simulink model "ES_video_newton_DSAS"  (R2020a)
settings: Solver=ode2  StartTime=0.0  StopTime=100  FixedStep=1/120  RelTol=1e-3
model workspace (MAT data in the model file):
  camera_rate = Simulink.Parameter
  camera_rate.Value = Simulink.data.Expression
  camera_rate.Value.ExpressionString = "qc_get_step_size * ceil(1/120 / qc_get_step_size)"
  camera_rate.DataType = 'auto'
  camera_rate.Dimensions = -1
  depth_rate = Simulink.Parameter
  depth_rate.Value = Simulink.data.Expression
  depth_rate.Value.ExpressionString = "qc_get_step_size * ceil(1/100 / qc_get_step_size)"
  depth_rate.DataType = 'auto'
  depth_rate.Dimensions = -1
values from neighbouring files (symbols this model uses):
  a_min = 0.01*[2;3;2;3;5;2]    [Parameters.m]
  amp = 0.5*[2;3;4;3;5;2]    [Parameters.m]
  d = 10*ones(6,1)    [Parameters.m]
  freq = 0.8*[0.0011;0.0054;0.0023;0.0037;0.0082;0.0041]*100    [Parameters.m]
  gain = (5*[30;20;21;10;15;20])    [Parameters.m]
  gain_amp = 0.001*[1;1;1;1;1;1]    [Parameters.m]
  IC = 1/2*diag([1 1 1 1 1 1])    [Parameters.m]
  r = 0.5    [Parameters.m]
  w_r = w * delta * 1    (= 0.01)    [Parameters.m]
undefined symbols (not defined in the file or in its folder): gcbh, JPEG, qc_get_step_size, video_display_show
libraries: quarc_library x13, simulink x3, powerlib_meascontrol x2, dspstat3 x1, visionsources x1
settings Model: PacingRate=8  ExtModeTrigDuration=10000  Creator=User  LastModifiedBy=user
settings SolverCC: PositivePriorityOrder=on
settings DataIOCC: ReturnWorkspaceOutputs=off
settings DebuggingCC: ParameterPrecisionLossMsg=none  ArithmeticOperatorsInVariantConditions=warning
settings HardwareCC: ProdBitPerLong=64  ProdLargestAtomicInteger=LongLong  ProdLargestAtomicFloat=Double  ProdLongLongMode=on  ProdHWDeviceType=ARM Compatible->ARM 64-bit (LP64)
settings SFSimCC: SimUseLocalCustomCode=off  CustomCodeUndefinedFunction=UseInterfaceOnly
settings RTWCC: Description=QUARC Linux Nvidia Target (QCar) Using Toolchain  SystemTargetFile=quarc_linux_nvidia.tlc  TemplateMakefile=quarc_default_tmf  RTWUseLocalCustomCode=off  Toolchain=QUARC linux_nvidia | gmake (64-bit Windows)  BuildConfiguration=Faster Runs
settings STFCustomTargetCC: TargetLangStandard=C99 (ISO)  ConcurrentExecutionCompliant=on  GRTInterface=on  UseToolchainInfoCompliant=on  SystemTargetFile=quarc_linux_nvidia.tlc
settings GRTTargetCC: ParMdlRefBuildCompliant=off  CompOptLevelCompliant=off  CombineOutputUpdateFcns=off  MatFileLogging=off  CPPClassGenCompliant=off  GRTInterface=on  ExtMode=on  ExtModeMexFile=quarc_comm  ExtModeMexArgs='-w -d /tmp -uri %u', 'tcpip://192.168.2.11:17001'

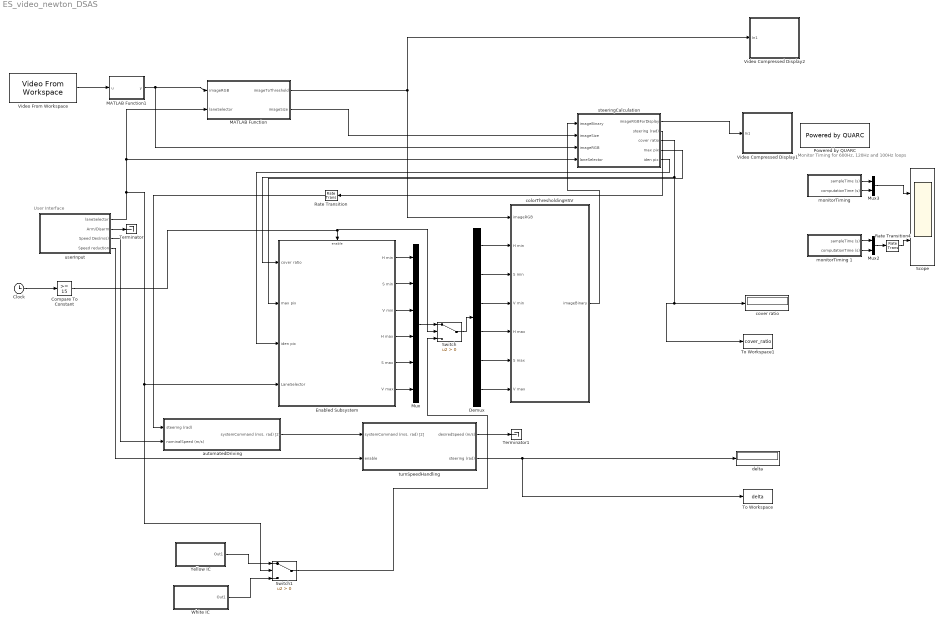
== system ES_video_newton_DSAS ==
  note: User Interface
  note: Monitor Timing for 600Hz, 120Hz and 100Hz loops
  Clock : Clock
  Compare To Constant : simulink/Logic and Bit Operations/Compare To Constant  relop=>=  const=15  OutDataTypeStr=boolean
  Demux : Demux  Outputs=6
  Enabled Subsystem : Subsystem  TreatAsAtomicUnit=on
  MATLAB Function : MATLAB Function  TreatAsAtomicUnit=on
  MATLAB Function1 : MATLAB Function  TreatAsAtomicUnit=on
  Mux : Mux  Inputs=6
  Mux2 : Mux  Inputs=2
  Mux3 : Mux  Inputs=2
  Powered by QUARC : quarc_library/Logos/Powered by QUARC
  Rate Transition : RateTransition
  Rate Transition4 : RateTransition
  Scope : Scope  NumInputPorts=2
  Switch : Switch  Criteria=u2 > Threshold
  Switch1 : Switch  Criteria=u2 > Threshold
  Terminator : Terminator
  Terminator1 : Terminator
  To Workspace : ToWorkspace  VariableName=delta  SaveFormat=Structure With Time  SampleTime=-1
  To Workspace1 : ToWorkspace  VariableName=cover_ratio  SaveFormat=Structure With Time  SampleTime=-1
      settings: Save2DSignal=2-D array (concatenate along first dimension)
  Video Compressed Display1 : Subsystem  LoadFcn=set_param(gcbh, 'UserData', gcb);  StartFcn=video_display_show([gcb, '/Video Display'], 'add', gcb);  mask(Video Compressed Display){algorithm=JPEG, quality=50, sample_time=-1, use_hardware=on}
      mask prompts: algorithm "Compression algorithm:"; quality "Compression quality (0-100):"; sample_time "Sample time (seconds):"; use_hardware "Use hardware acceleration for video display"
      mask help: Displays a video stream on the host, using compression to minimize bandwidth.
      mask init:
      | qc_set_display('Video\nCompressed\nDisplay');
      settings: UndoDeleteFcn=set_param(gcbh, 'UserData', gcb);  OpenFcn=video_display_show([gcb, '/Video Display'], 'show', gcb);  PreDeleteFcn=video_display_show([gcb, '/Video Display'], 'delete');
      settings: CopyFcn=|
      | set_param(gcbh, 'UserData', gcb);
      | set_param(gcbh, 'LinkStatus', 'none');
      settings: NameChangeFcn=|
      | video_display_show([get_param(gcbh, 'UserData'), '/Video Display'], 'rename', [gcb, '/Video Display']);
      | video_display_show([gcb, '/Video Display'], 'add', gcb);
      | set_param(gcbh, 'UserData', gcb);
      mask Help: web(qc_get_block_help_path(gcb));
      mask TypeOptions algorithm: Image Compress/algorithm
      mask TypeOptions quality: Image Compress/quality
      mask TypeOptions sample_time: Video Display/sample_time
      mask TypeOptions use_hardware: Video Display/use_hardware
      mask Display:
      | patch([0.98591 0.98591 0.62618 0.59072 0.56147   0.536   0.536  0.5441 0.56912 0.59207 0.60881 0.62276 0.63527 0.64364  0.6485  0.6485 0.64706 0.64499 0.63662 0.62411 0.61232 0.59837 0.58307 0.56147   0.536   0.536  0.5441  0.5747 0.60953 0.63662 0.67001  0.7034 0.72851 0.75425 0.77927 0.80294 0.82454 0.84119 0.85865 0.87395 0.88574 0.89339  0.8969 0.89969 0.89969 0.89267  0.8816 0.87044 0.85649  0.8384 0.81824 0.80294 0.78764 0.77513 0.76676 0.75776 0.76397 0.77513 0.79178 0.80987 0.82796 0.84326 0.86207 0.98528],[0.18689 0.05522 0.05522 0.05171 0.05171    0.05 0.18338 0.18338 0.19148 0.20435 0.22298 0.24863 0.28589 0.33125 0.38138 0.55139 0.59801 0.63761 0.68189 0.72149 0.74939 0.76694 0.77855 0.79367 0.79952 0.92768 0.92768 0.92768 0.92417 0.92066 0.91364  0.9032 0.89384 0.88106 0.86594 0.85073 0.82634 0.80537 0.77855 0.74363 0.70403 0.65858 0.61079 0.59099 0.41513 0.37202 0.31847 0.29048 0.25556 0.23342  0.2102 0.19382 0.18221 0.17285 0.16943 0.16124  0.1589 0.16241 0.16709 0.17168  0.1787 0.18221 0.18689 0.18689],[0.9,0.90,0.91])
      | patch([0.536 0.52601 0.46823 0.44528 0.41603 0.39101 0.35555 0.33116 0.31451 0.29291  0.2804 0.26717 0.25322 0.23999 0.22406 0.20732 0.19337 0.17528 0.15935 0.14396 0.13217 0.11759 0.10922 0.10085 0.09671 0.09392 0.09041 0.08906 0.08906 0.09464  0.0995 0.10778 0.11894 0.13145 0.14675 0.16349 0.17672 0.19409 0.20732 0.22406 0.23999 0.26159 0.27833 0.29849 0.31793 0.33602 0.35411 0.37085 0.39245 0.41603   0.536   0.536 0.53159 0.46409   0.446 0.42026 0.39587 0.37571 0.36113 0.34925 0.34088 0.33809 0.33809 0.34088 0.34583 0.35627 0.36392 0.38129 0.39587 0.41117 0.42719 0.44672  0.4676 0.48353 0.48353 0.52394   0.536],[0.05 0.04829 0.04712 0.04712 0.04829 0.05063 0.05405 0.05873 0.06107 0.06692 0.07043 0.07619 0.08087 0.08672 0.09482 0.10652 0.11696 0.13325  0.1508 0.17168 0.19499 0.22415 0.25439 0.28472 0.31379 0.35456 0.38489 0.41513 0.58055 0.63878 0.68774 0.72149 0.75641 0.78089 0.80537 0.82859 0.84029 0.85658 0.86594 0.87404  0.8834 0.89267 0.90086 0.90788 0.91247 0.91832 0.92066   0.923 0.92651 0.92768 0.92768 0.79952 0.79952 0.79952 0.79718 0.78899 0.77153 0.75056 0.72149 0.68072 0.62249  0.5549 0.41396 0.37085 0.33242 0.28121 0.25205 0.22181 0.20552 0.19499 0.18572 0.18221 0.17753 0.17636 0.17753  0.1787  0.1787],[0.9,0.90,0.91])
      | disp('Video\nCompressed\nDisplay');
  Video Compressed Display2 : Subsystem  LoadFcn=set_param(gcbh, 'UserData', gcb);  StartFcn=video_display_show([gcb, '/Video Display'], 'add', gcb);  mask(Video Compressed Display){algorithm=JPEG, quality=50, sample_time=-1, use_hardware=on}
      mask prompts: algorithm "Compression algorithm:"; quality "Compression quality (0-100):"; sample_time "Sample time (seconds):"; use_hardware "Use hardware acceleration for video display"
      mask help: Displays a video stream on the host, using compression to minimize bandwidth.
      mask init:
      | qc_set_display('Video\nCompressed\nDisplay');
      settings: UndoDeleteFcn=set_param(gcbh, 'UserData', gcb);  OpenFcn=video_display_show([gcb, '/Video Display'], 'show', gcb);  PreDeleteFcn=video_display_show([gcb, '/Video Display'], 'delete');
      settings: CopyFcn=|
      | set_param(gcbh, 'UserData', gcb);
      | set_param(gcbh, 'LinkStatus', 'none');
      settings: NameChangeFcn=|
      | video_display_show([get_param(gcbh, 'UserData'), '/Video Display'], 'rename', [gcb, '/Video Display']);
      | video_display_show([gcb, '/Video Display'], 'add', gcb);
      | set_param(gcbh, 'UserData', gcb);
      mask Help: web(qc_get_block_help_path(gcb));
      mask TypeOptions algorithm: Image Compress/algorithm
      mask TypeOptions quality: Image Compress/quality
      mask TypeOptions sample_time: Video Display/sample_time
      mask TypeOptions use_hardware: Video Display/use_hardware
      mask Display:
      | patch([0.98591 0.98591 0.62618 0.59072 0.56147   0.536   0.536  0.5441 0.56912 0.59207 0.60881 0.62276 0.63527 0.64364  0.6485  0.6485 0.64706 0.64499 0.63662 0.62411 0.61232 0.59837 0.58307 0.56147   0.536   0.536  0.5441  0.5747 0.60953 0.63662 0.67001  0.7034 0.72851 0.75425 0.77927 0.80294 0.82454 0.84119 0.85865 0.87395 0.88574 0.89339  0.8969 0.89969 0.89969 0.89267  0.8816 0.87044 0.85649  0.8384 0.81824 0.80294 0.78764 0.77513 0.76676 0.75776 0.76397 0.77513 0.79178 0.80987 0.82796 0.84326 0.86207 0.98528],[0.18689 0.05522 0.05522 0.05171 0.05171    0.05 0.18338 0.18338 0.19148 0.20435 0.22298 0.24863 0.28589 0.33125 0.38138 0.55139 0.59801 0.63761 0.68189 0.72149 0.74939 0.76694 0.77855 0.79367 0.79952 0.92768 0.92768 0.92768 0.92417 0.92066 0.91364  0.9032 0.89384 0.88106 0.86594 0.85073 0.82634 0.80537 0.77855 0.74363 0.70403 0.65858 0.61079 0.59099 0.41513 0.37202 0.31847 0.29048 0.25556 0.23342  0.2102 0.19382 0.18221 0.17285 0.16943 0.16124  0.1589 0.16241 0.16709 0.17168  0.1787 0.18221 0.18689 0.18689],[0.9,0.90,0.91])
      | patch([0.536 0.52601 0.46823 0.44528 0.41603 0.39101 0.35555 0.33116 0.31451 0.29291  0.2804 0.26717 0.25322 0.23999 0.22406 0.20732 0.19337 0.17528 0.15935 0.14396 0.13217 0.11759 0.10922 0.10085 0.09671 0.09392 0.09041 0.08906 0.08906 0.09464  0.0995 0.10778 0.11894 0.13145 0.14675 0.16349 0.17672 0.19409 0.20732 0.22406 0.23999 0.26159 0.27833 0.29849 0.31793 0.33602 0.35411 0.37085 0.39245 0.41603   0.536   0.536 0.53159 0.46409   0.446 0.42026 0.39587 0.37571 0.36113 0.34925 0.34088 0.33809 0.33809 0.34088 0.34583 0.35627 0.36392 0.38129 0.39587 0.41117 0.42719 0.44672  0.4676 0.48353 0.48353 0.52394   0.536],[0.05 0.04829 0.04712 0.04712 0.04829 0.05063 0.05405 0.05873 0.06107 0.06692 0.07043 0.07619 0.08087 0.08672 0.09482 0.10652 0.11696 0.13325  0.1508 0.17168 0.19499 0.22415 0.25439 0.28472 0.31379 0.35456 0.38489 0.41513 0.58055 0.63878 0.68774 0.72149 0.75641 0.78089 0.80537 0.82859 0.84029 0.85658 0.86594 0.87404  0.8834 0.89267 0.90086 0.90788 0.91247 0.91832 0.92066   0.923 0.92651 0.92768 0.92768 0.79952 0.79952 0.79952 0.79718 0.78899 0.77153 0.75056 0.72149 0.68072 0.62249  0.5549 0.41396 0.37085 0.33242 0.28121 0.25205 0.22181 0.20552 0.19499 0.18572 0.18221 0.17753 0.17636 0.17753  0.1787  0.1787],[0.9,0.90,0.91])
      | disp('Video\nCompressed\nDisplay');
  Video From Workspace : visionsources/Video From Workspace  signal=led  Ts=1/12  finalout=Obsolete  finaloutActive=Setting to zero  imagePorts=One multidimensional signal  OutPortLabels=R|G|B
      settings: SourceProductBaseCode=VP
  White IC : Subsystem
  Yellow IC : Subsystem
  automatedDriving : Subsystem
  colorThresholdingHSV : Subsystem
  cover ratio : Display
  "delta " : Display
  "monitorTiming " : Subsystem
  monitorTiming 1 : Subsystem
  steeringCalculation : Subsystem
  turnSpeedHandling : Subsystem
  userInput : Subsystem
  wires:
  userInput/4(Speed reduction) -> turnSpeedHandling/2(enable)
  automatedDriving/1("systemCommand (m/s, rad) [2]") -> turnSpeedHandling/1("systemCommand (m/s, rad) [2]")
  Rate Transition/1 -> automatedDriving/1(steering (rad))
  monitorTiming 1/2(computationTime (s)) -> Mux2/2
  monitorTiming 1/1(sampleTime (s)) -> Mux2/1
  "monitorTiming "/2(computationTime (s)) -> Mux3/2
  "monitorTiming "/1(sampleTime (s)) -> Mux3/1
  Mux2/1 -> Rate Transition4/1
  Mux3/1 -> Scope/1
  Rate Transition4/1 -> Scope/2
  colorThresholdingHSV/1(imageBinary) -> steeringCalculation/1(imageBinary)
  steeringCalculation/1(imageRGBForDisplay) -> Video Compressed Display1/1(In1)
  MATLAB Function/1(imageToThreshold) -> Video Compressed Display2/1(In1), colorThresholdingHSV/1(imageRGB)
  MATLAB Function/2(imageSize) -> steeringCalculation/2(imageSize)
  userInput/3(Speed Des(m/s)) -> automatedDriving/2(nominalSpeed (m/s))
  steeringCalculation/2(steering (rad)) -> Rate Transition/1
  Video From Workspace/1 -> MATLAB Function1/1(u)
  userInput/2(Arm/Disarm) -> Terminator/1
  MATLAB Function1/1(y) -> steeringCalculation/3(imageRGB), MATLAB Function/1(imageRGB)
  turnSpeedHandling/2(steering (rad)) -> To Workspace/1, "delta "/1
  steeringCalculation/3("cover ratio ") -> Enabled Subsystem/1(cover ratio), To Workspace1/1, cover ratio/1
  turnSpeedHandling/1(desiredSpeed (m/s)) -> Terminator1/1
  Clock/1 -> Compare To Constant/1
  Compare To Constant/1 -> Switch/2, Enabled Subsystem/Enable
  Enabled Subsystem/1(H min) -> Mux/1
  Enabled Subsystem/2(S min) -> Mux/2
  Enabled Subsystem/3(V min) -> Mux/3
  Enabled Subsystem/4(H max) -> Mux/4
  Enabled Subsystem/5(S max) -> Mux/5
  Enabled Subsystem/6(V max) -> Mux/6
  Mux/1 -> Switch/1
  Demux/6 -> colorThresholdingHSV/7(V max)
  Switch/1 -> Demux/1
  Demux/1 -> colorThresholdingHSV/2(H min)
  Demux/2 -> colorThresholdingHSV/3(S min)
  Demux/3 -> colorThresholdingHSV/4(V min)
  Demux/4 -> colorThresholdingHSV/5(H max)
  Demux/5 -> colorThresholdingHSV/6(S max)
  steeringCalculation/4(max pix) -> Enabled Subsystem/2(max pix)
  steeringCalculation/5(iden pix) -> Enabled Subsystem/3(iden pix)
  White IC/1(Out1) -> Switch1/3
  Yellow IC/1(Out1) -> Switch1/1
  Switch1/1 -> Switch/3
  userInput/1(laneSelector) -> Enabled Subsystem/4(LaneSelector), Switch1/2, MATLAB Function/2(laneSelector), steeringCalculation/4(laneSelector)

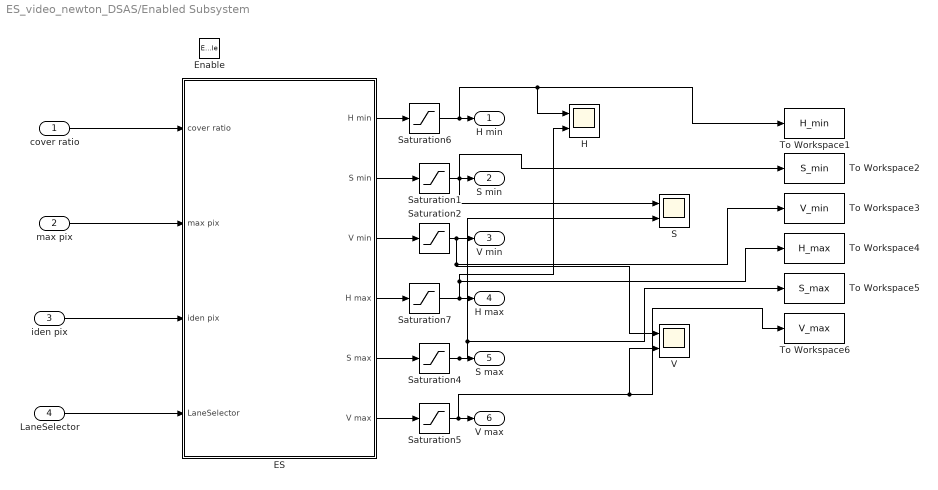
== system ES_video_newton_DSAS/Enabled Subsystem ==
  cover ratio : Inport
  max pix : Inport  Port=2
  iden pix : Inport  Port=3
  LaneSelector : Inport  Port=4
  Enable : EnablePort
  ES : Subsystem
  H : Scope  NumInputPorts=2
  S : Scope  NumInputPorts=2
  Saturation{1..2,4..7} (6 alike) : Saturate  UpperLimit=255  LowerLimit=0
  To Workspace1 : ToWorkspace  VariableName=H_min  SaveFormat=Timeseries  SampleTime=-1
      settings: Save2DSignal=2-D array (concatenate along first dimension)
  To Workspace2 : ToWorkspace  VariableName=S_min  SaveFormat=Timeseries  SampleTime=-1
      settings: Save2DSignal=2-D array (concatenate along first dimension)
  To Workspace3 : ToWorkspace  VariableName=V_min  SaveFormat=Timeseries  SampleTime=-1
      settings: Save2DSignal=2-D array (concatenate along first dimension)
  To Workspace4 : ToWorkspace  VariableName=H_max  SaveFormat=Timeseries  SampleTime=-1
      settings: Save2DSignal=2-D array (concatenate along first dimension)
  To Workspace5 : ToWorkspace  VariableName=S_max  SaveFormat=Timeseries  SampleTime=-1
      settings: Save2DSignal=2-D array (concatenate along first dimension)
  To Workspace6 : ToWorkspace  VariableName=V_max  SaveFormat=Timeseries  SampleTime=-1
      settings: Save2DSignal=2-D array (concatenate along first dimension)
  V : Scope  NumInputPorts=2
  H min : Outport  VectorParamsAs1DForOutWhenUnconnected=off
  S min : Outport  Port=2  VectorParamsAs1DForOutWhenUnconnected=off
  V min : Outport  Port=3  VectorParamsAs1DForOutWhenUnconnected=off
  H max : Outport  Port=4  VectorParamsAs1DForOutWhenUnconnected=off
  S max : Outport  Port=5  VectorParamsAs1DForOutWhenUnconnected=off
  V max : Outport  Port=6  VectorParamsAs1DForOutWhenUnconnected=off
  wires:
  cover ratio/1 -> ES/1("cover ratio ")
  ES/2(S min) -> Saturation1/1
  ES/3(V min) -> Saturation2/1
  ES/5(S max) -> Saturation4/1
  ES/6(V max) -> Saturation5/1
  max pix/1 -> ES/2("max pix ")
  iden pix/1 -> ES/3(iden pix)
  Saturation2/1 -> To Workspace3/1, V/1, V min/1
  Saturation5/1 -> To Workspace6/1, V/2, V max/1
  ES/4(H max) -> Saturation7/1
  Saturation1/1 -> To Workspace2/1, S min/1, S/1
  Saturation4/1 -> To Workspace5/1, S/2, S max/1
  ES/1(H min) -> Saturation6/1
  Saturation6/1 -> To Workspace1/1, H/1, H min/1
  Saturation7/1 -> To Workspace4/1, H/2, H max/1
  LaneSelector/1 -> ES/4(LaneSelector)

== system ES_video_newton_DSAS/Video Compressed Display1 ==
  In1 : Inport
  Channel : quarc_library/Signal Routing/Channel  channel=0  buffer_size=1
  Image Compress : quarc_library/Image Processing/Generic/Image Compress  algorithm=JPEG  source=Internal dialog parameter  quality=quality  output_dim=-1
  Video Display : quarc_library/Multimedia/Video Display  Tag=ES_video_newton_DSAS/Video Compressed Display1/Video Display  sample_time=sample_time  use_hardware=on
  wires:
  Channel/1 -> Video Display/1
  In1/1 -> Image Compress/1
  Image Compress/1 -> Channel/1

== system ES_video_newton_DSAS/Video Compressed Display2 ==
  In1 : Inport
  Channel : quarc_library/Signal Routing/Channel  channel=1  buffer_size=1
  Image Compress : quarc_library/Image Processing/Generic/Image Compress  algorithm=JPEG  source=Internal dialog parameter  quality=quality  output_dim=-1
  Video Display : quarc_library/Multimedia/Video Display  Tag=ES_video_newton_DSAS/Video Compressed Display2/Video Display  sample_time=sample_time  use_hardware=on
  wires:
  Image Compress/1 -> Channel/1
  In1/1 -> Image Compress/1
  Channel/1 -> Video Display/1

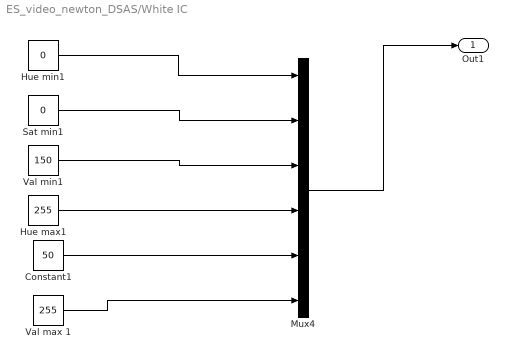
== system ES_video_newton_DSAS/White IC ==
  Constant1 : Constant  Value=50
  Hue max1 : Constant  Value=255
  Hue min1 : Constant  Value=0
  Mux4 : Mux  Inputs=6
  Sat min1 : Constant  Value=0
  Val max 1 : Constant  Value=255
  Val min1 : Constant  Value=150
  Out1 : Outport  VectorParamsAs1DForOutWhenUnconnected=off
  wires:
  Mux4/1 -> Out1/1
  Constant1/1 -> Mux4/5
  Sat min1/1 -> Mux4/2
  Hue min1/1 -> Mux4/1
  Val min1/1 -> Mux4/3
  Val max 1/1 -> Mux4/6
  Hue max1/1 -> Mux4/4

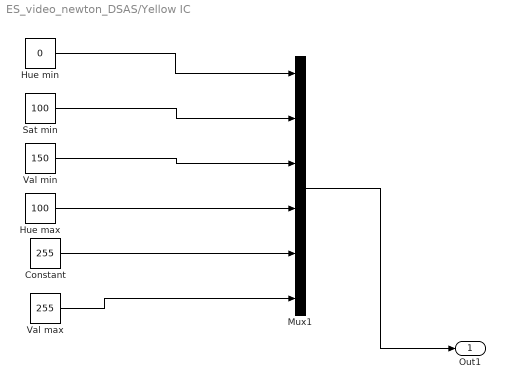
== system ES_video_newton_DSAS/Yellow IC ==
  Constant : Constant  Value=255
  Hue max : Constant  Value=100
  Hue min : Constant  Value=0
  Mux1 : Mux  Inputs=6
  Sat min : Constant  Value=100
  "Val max " : Constant  Value=255
  Val min : Constant  Value=150
  Out1 : Outport  VectorParamsAs1DForOutWhenUnconnected=off
  wires:
  Hue max/1 -> Mux1/4
  Val min/1 -> Mux1/3
  Hue min/1 -> Mux1/1
  "Val max "/1 -> Mux1/6
  Mux1/1 -> Out1/1
  Constant/1 -> Mux1/5
  Sat min/1 -> Mux1/2

== system ES_video_newton_DSAS/automatedDriving ==
  note: Automated-Driving Module:
      |
      | This subsystem provides a speed setpoint based on obstacles detected, while also transitioning rates. The speed setpoint is set to the nominal speed, and scales down linearly to zero depending on nominal tracking distance and stop distance.
      |
      | Inputs:
      | obstacleDistance (m) n/a : Distance to obstacle in meters
      | steering (rad) n/a : Steering output from image processing in radians
      | nominalSpeed (m/s) n/a : Desired speed setpoint
      |
      | Outputs:
      | systemCommand (m/s, rad) n/a : Commands representing speed setpoint and steering
      |
      | Usage:
      | 1. Set the Nominal Tracking distance. The speed setpoint will start decreasing if the obstacle distance is less than this threshold.
      | 2. Set the Stop Distance. The speed setpoint will scale down to 0 when the the obstacle distance reaches this threshold.
  steering (rad) : Inport
  nominalSpeed (m/s) : Inport  Port=2
  Mux1 : Mux  Inputs=2
  "systemCommand (m/s, rad) [2]" : Outport  VectorParamsAs1DForOutWhenUnconnected=off
  wires:
  nominalSpeed (m/s)/1 -> Mux1/1  "nominal speed (m/s)"
  steering (rad)/1 -> Mux1/2
  Mux1/1 -> "systemCommand (m/s, rad) [2]"/1

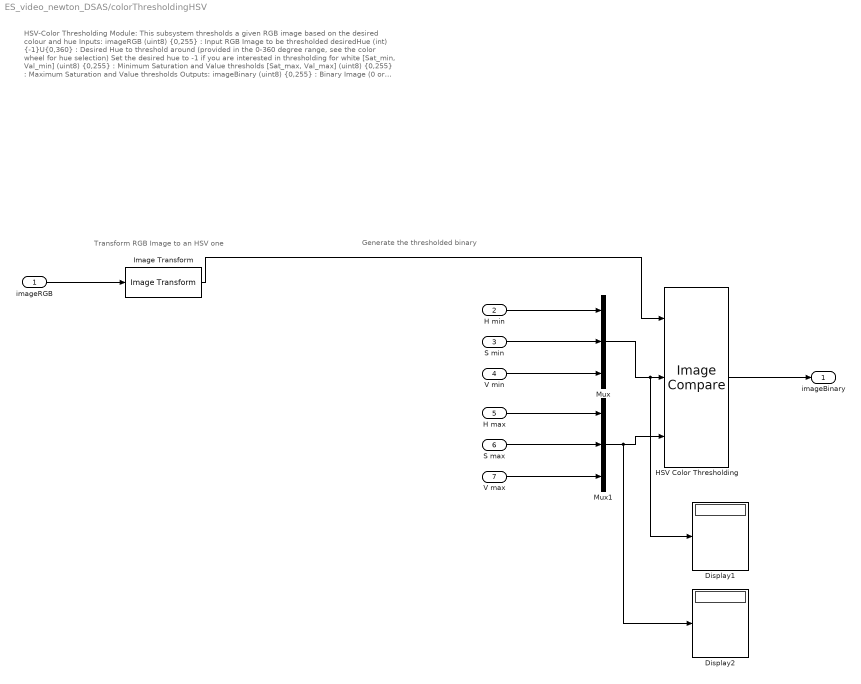
== system ES_video_newton_DSAS/colorThresholdingHSV ==
  note: HSV-Color Thresholding Module:
      |
      | This subsystem thresholds a given RGB image based on the desired colour and hue
      |
      | Inputs:
      | imageRGB (uint8) {0,255} : Input RGB Image to be thresholded
      | desiredHue (int) {-1}U{0,360} : Desired Hue to threshold around (provided in the 0-360 degree range, see the color wheel for hue selection)
      | Set the desired hue to -1 if you are interested in thresholding for white
      | [Sat_min, Val_min] (uint8) {0,255} : Minimum Saturation and Value thresholds
      | [Sat_max, Val_max] (uint8) {0,255} : Maximum Saturation and Value thresholds
      |
      | Outputs:
      | imageBinary (uint8) {0,255} : Binary Image (0 or 255 and no other value) representing the thresholding output
      |
      | Usage:
      | This module can be used when you are interested in thresholding for a certain hue regardless of the luminance. Compared to RGB thresholding which does not work well when the lighting conditions vary, HSV thresholding will correctly threshold for a hue (color) and allow you to specify a broad range of illuminance via the saturation and value thresholds. To broaden the range of hues accepted in the thresholding block, increase the Hue Threshold parameter.
  note: Transform RGB Image to an HSV one
  note: Generate the thresholded binary
  imageRGB : Inport
  H min : Inport  Port=2
  S min : Inport  Port=3
  V min : Inport  Port=4
  H max : Inport  Port=5
  S max : Inport  Port=6
  V max : Inport  Port=7
  Display1 : Display
  Display2 : Display
  HSV Color Thresholding : quarc_library/Image Processing/Generic/Image Compare  output_type=Combined (one HxW output)  source=External input ports  r_comparison=min <= pixel and pixel <= max with wrapping  r_minimum=30  r_maximum=70  g_comparison=min <= pixel and pixel <= max with wrapping  g_minimum=60  g_maximum=100  b_comparison=min <= pixel and pixel <= max with wrapping  b_minimum=40  b_maximum=80
      settings: SourceProductName=QUARC Targets
  Image Transform : quarc_library/Image Processing/Generic/Image Transform  algorithm=RGB to HSV  color_theme=KRYGCBMW  min_pixel=0  max_pixel=4000  focal_length=308  principal_point=[334 262]  radial_coeffs=[-0.3129 0.0907]  tangential_coeffs=[]  extrapolated_pixel=0  interpolation=nearest  row_coords=0  column_coords=0  output_height=480  output_width=640  angle=0  origin=[320 240]  output_origin=[320 240]
      settings: AttributesFormatString=(%<algorithm>)  SourceProductName=QUARC Targets
  Mux : Mux  Inputs=3
  Mux1 : Mux  Inputs=3
  imageBinary : Outport  VectorParamsAs1DForOutWhenUnconnected=off
  wires:
  Image Transform/1 -> HSV Color Thresholding/1
  imageRGB/1 -> Image Transform/1
  HSV Color Thresholding/1 -> imageBinary/1
  Mux/1 -> Display1/1, HSV Color Thresholding/2
  Mux1/1 -> Display2/1, HSV Color Thresholding/3
  S min/1 -> Mux/2
  H max/1 -> Mux1/1
  S max/1 -> Mux1/2
  V max/1 -> Mux1/3
  H min/1 -> Mux/1
  V min/1 -> Mux/3

== system ES_video_newton_DSAS/monitorTiming  ==
  note: moniorTiming Module:
      |
      | This subsystem outputs the sample time and computation time of the model.
      |
      | Outputs:
      | sampleTime (s) n/a : Sample time (unfiltered and filtered) in seconds.
      | computationTime (s) n/a : Computation time (unfiltered and filtered) in seconds.
      |
      | Usage:
      | Compare the Sample Time (s) output to a constant (qc_get_step_size) to monitor whether or not the desired sample time is being achieved. The Computation Time (s) values should be lower than the corresponding sample time value to ensure that the solver has enough time per time step.
  note: Timing Performance
  Computation Time : quarc_library/Sources/Time/Computation Time  sample_time=qc_get_step_size  use_model=on  use_cpu_time=off
  Constant : Constant  Value=qc_get_step_size  SampleTime=-1
  Mux : Mux  Inputs=2
  Sample Time : quarc_library/Sources/Time/Sample Time  Priority=-99  sample_time=qc_get_step_size
  sampleTime (s) : Outport  VectorParamsAs1DForOutWhenUnconnected=off
  computationTime (s) : Outport  Port=2  VectorParamsAs1DForOutWhenUnconnected=off
  wires:
  Computation Time/1 -> computationTime (s)/1
  Constant/1 -> Mux/2
  Sample Time/1 -> Mux/1
  Mux/1 -> sampleTime (s)/1

== system ES_video_newton_DSAS/monitorTiming 1 ==
  note: Timing Performance
  note: moniorTiming Module:
      |
      | This subsystem outputs the sample time and computation time of the model.
      |
      | Outputs:
      | sampleTime (s) n/a : Sample time (unfiltered and filtered) in seconds.
      | computationTime (s) n/a : Computation time (unfiltered and filtered) in seconds.
      |
      | Usage:
      | Compare the Sample Time (s) output to a constant (qc_get_step_size) to monitor whether or not the desired sample time is being achieved. The Computation Time (s) values should be lower than the corresponding sample time value to ensure that the solver has enough time per time step.
  Computation Time : quarc_library/Sources/Time/Computation Time  sample_time=camera_rate  use_model=on  use_cpu_time=off
  Constant : Constant  Value=camera_rate  SampleTime=camera_rate
  Mux : Mux  Inputs=2
  Sample Time : quarc_library/Sources/Time/Sample Time  Priority=-99  sample_time=camera_rate
  sampleTime (s) : Outport  VectorParamsAs1DForOutWhenUnconnected=off
  computationTime (s) : Outport  Port=2  VectorParamsAs1DForOutWhenUnconnected=off
  wires:
  Computation Time/1 -> computationTime (s)/1
  Mux/1 -> sampleTime (s)/1
  Sample Time/1 -> Mux/1
  Constant/1 -> Mux/2

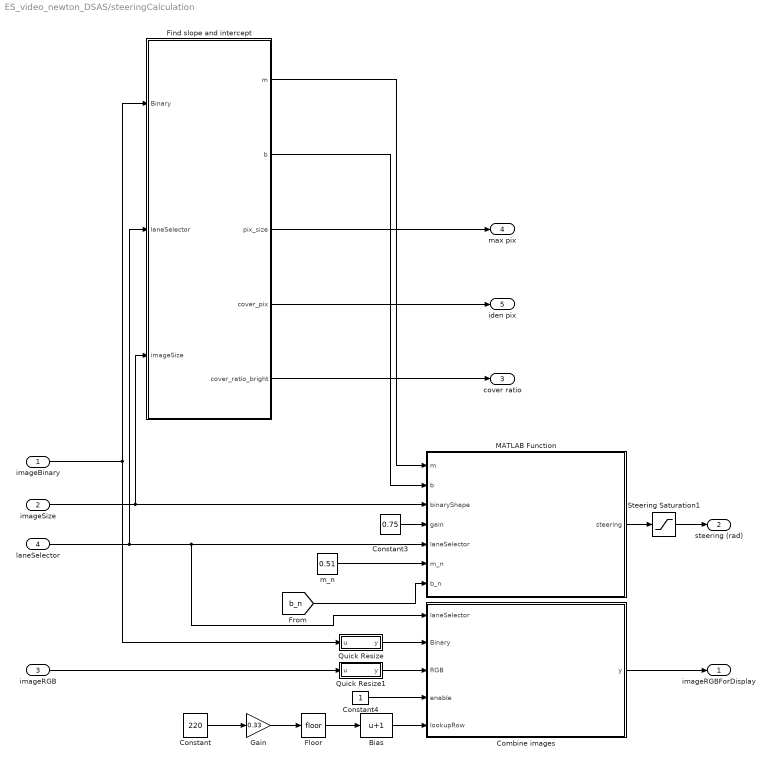
== system ES_video_newton_DSAS/steeringCalculation ==
  imageBinary : Inport
  imageSize : Inport  Port=2
  imageRGB : Inport  Port=3
  laneSelector : Inport  Port=4
  Bias : Bias  Bias=1
  Combine images : MATLAB Function  TreatAsAtomicUnit=on
  Constant : Constant  Value=220
  Constant3 : Constant  Value=0.75
  Constant4 : Constant
  Find slope and intercept : MATLAB Function  TreatAsAtomicUnit=on
  Floor : Rounding
  Gain : Gain  Gain=0.33
  MATLAB Function : MATLAB Function  TreatAsAtomicUnit=on
  Quick Resize : MATLAB Function  TreatAsAtomicUnit=on
  Quick Resize1 : MATLAB Function  TreatAsAtomicUnit=on
  Steering Saturation1 : Saturate
  m_n : Constant  Value=0.51
  imageRGBForDisplay : Outport  VectorParamsAs1DForOutWhenUnconnected=off
  steering (rad) : Outport  Port=2  VectorParamsAs1DForOutWhenUnconnected=off
  "cover ratio " : Outport  Port=3  VectorParamsAs1DForOutWhenUnconnected=off
  max pix : Outport  Port=4  VectorParamsAs1DForOutWhenUnconnected=off
  iden pix : Outport  Port=5  VectorParamsAs1DForOutWhenUnconnected=off
  wires:
  Find slope and intercept/1(m) -> MATLAB Function/1(m)
  laneSelector/1 -> MATLAB Function/5(laneSelector), Combine images/1(laneSelector), Find slope and intercept/2(laneSelector)
  MATLAB Function/1(steering) -> Steering Saturation1/1
  Constant3/1 -> MATLAB Function/4(gain)
  imageBinary/1 -> Quick Resize/1(u), Find slope and intercept/1(Binary)
  Find slope and intercept/2(b) -> MATLAB Function/2(b)
  Constant4/1 -> Combine images/4(enable)
  Quick Resize/1(y) -> Combine images/2(Binary)
  Quick Resize1/1(y) -> Combine images/3(RGB)
  Combine images/1(y) -> imageRGBForDisplay/1
  imageRGB/1 -> Quick Resize1/1(u)
  Steering Saturation1/1 -> steering (rad)/1
  Gain/1 -> Floor/1
  imageSize/1 -> MATLAB Function/3(binaryShape), Find slope and intercept/3(imageSize)
  Constant/1 -> Gain/1
  Bias/1 -> Combine images/5(lookupRow)
  Floor/1 -> Bias/1
  [b_n] -> MATLAB Function/7(b_n)
  m_n/1 -> MATLAB Function/6(m_n)
  Find slope and intercept/3(pix_size) -> max pix/1
  Find slope and intercept/4(cover_pix) -> iden pix/1
  Find slope and intercept/5(cover_ratio_bright) -> "cover ratio "/1

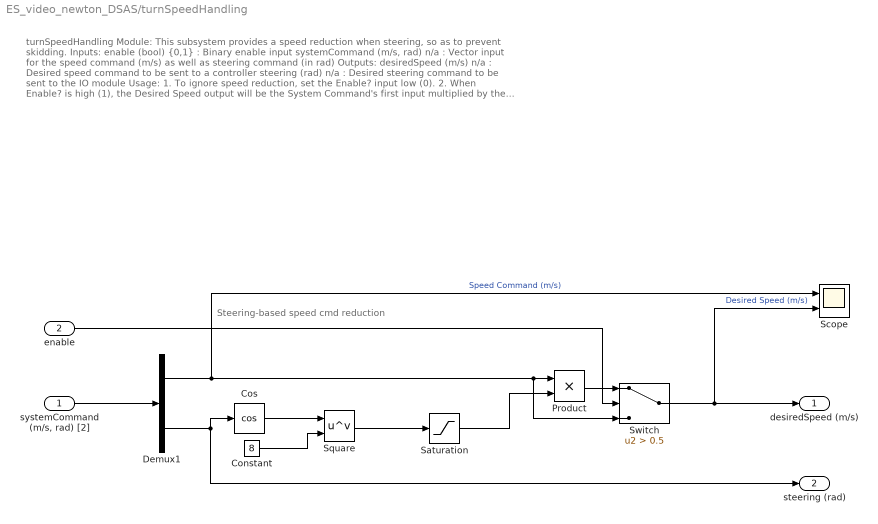
== system ES_video_newton_DSAS/turnSpeedHandling ==
  note: turnSpeedHandling Module:
      |
      | This subsystem provides a speed reduction when steering, so as to prevent skidding.
      |
      | Inputs:
      | enable (bool) {0,1} : Binary enable input
      | systemCommand (m/s, rad) n/a : Vector input for the speed command (m/s) as well as steering command (in rad)
      |
      | Outputs:
      | desiredSpeed (m/s) n/a : Desired speed command to be sent to a controller
      | steering (rad) n/a : Desired steering command to be sent to the IO module
      |
      | Usage:
      | 1. To ignore speed reduction, set the Enable? input low (0).
      | 2. When Enable? is high (1), the Desired Speed output will be the System Command's first input multiplied by the cosine of the steering. Note that the lower limit of this reduction is set to 50% of the speed command input.
  note: Steering-based speed cmd reduction
  "systemCommand (m/s, rad) [2]" : Inport
  enable : Inport  Port=2
  Constant : Constant  Value=8
  Cos : Trigonometry  Operator=cos
  Demux1 : Demux  Outputs=2
  Product : Product
  Saturation : Saturate  UpperLimit=1  LowerLimit=0.5
  Scope : Scope  NumInputPorts=2
  Square : Math  Operator=pow  SignedPower=on  SaturateOnIntegerOverflow=on
  Switch : Switch  Criteria=u2 > Threshold  Threshold=0.5
  desiredSpeed (m/s) : Outport  VectorParamsAs1DForOutWhenUnconnected=off
  steering (rad) : Outport  Port=2  VectorParamsAs1DForOutWhenUnconnected=off
  wires:
  Cos/1 -> Square/1
  Switch/1 -> desiredSpeed (m/s)/1, Scope/2  "Desired Speed (m/s)"
  Product/1 -> Switch/1
  Saturation/1 -> Product/2
  Demux1/1 -> Product/1, Switch/3, Scope/1  "Speed Command (m/s)"
  "systemCommand (m/s, rad) [2]"/1 -> Demux1/1
  enable/1 -> Switch/2
  Constant/1 -> Square/2
  Demux1/2 -> steering (rad)/1, Cos/1
  Square/1 -> Saturation/1

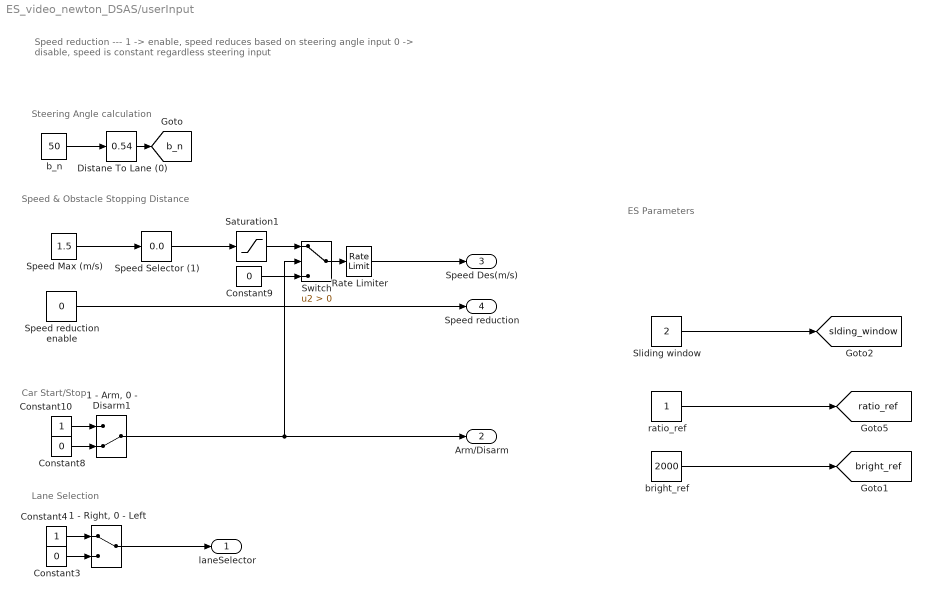
== system ES_video_newton_DSAS/userInput ==
  note: Speed reduction --- 1 -> enable, speed reduces based on steering angle input
      |                                 0 -> disable, speed is constant regardless steering input
  note: Lane Selection
  note: Car Start/Stop
  note: Steering Angle calculation
  note: Speed & Obstacle Stopping Distance
  note: ES Parameters
  "1 - Arm, 0 - Disarm1" : ManualSwitch  CurrentSetting=0
  "1 - Right, 0 - Left" : ManualSwitch
  Constant10 : Constant
  Constant3 : Constant  Value=0
  Constant4 : Constant
  Constant8 : Constant  Value=0
  Constant9 : Constant  Value=0
  "Distane To Lane (0) " : simulink/Math Operations/Slider Gain  gain=0.54  low=0  high=1
  Rate Limiter : RateLimiter  FallingSlewLimit=-Inf  SampleTimeMode=inherited
  Saturation1 : Saturate  UpperLimit=1  LowerLimit=0
  Sliding window : Constant  Value=2
  Speed Max (m/s) : Constant  Value=1.5
  Speed Selector (1) : simulink/Math Operations/Slider Gain  gain=0.0  low=0  high=1
  Speed reduction enable : Constant  Value=0
  Switch : Switch  Criteria=u2 > Threshold
  b_n : Constant  Value=50
  bright_ref : Constant  Value=2000
  ratio_ref : Constant
  laneSelector : Outport  VectorParamsAs1DForOutWhenUnconnected=off
  Arm/Disarm : Outport  Port=2  VectorParamsAs1DForOutWhenUnconnected=off
  Speed Des(m/s) : Outport  Port=3  VectorParamsAs1DForOutWhenUnconnected=off
  Speed reduction : Outport  Port=4  VectorParamsAs1DForOutWhenUnconnected=off
  tag scope: b_n=global, bright_ref=global, ratio_ref=global, slding_window=global
  wires:
  Constant3/1 -> "1 - Right, 0 - Left"/2
  "1 - Arm, 0 - Disarm1"/1 -> Switch/2, Arm/Disarm/1
  b_n/1 -> "Distane To Lane (0) "/1
  Constant4/1 -> "1 - Right, 0 - Left"/1
  Switch/1 -> Rate Limiter/1
  Constant9/1 -> Switch/3
  Speed Max (m/s)/1 -> Speed Selector (1)/1
  Saturation1/1 -> Switch/1
  Constant10/1 -> "1 - Arm, 0 - Disarm1"/1
  "1 - Right, 0 - Left"/1 -> laneSelector/1
  Rate Limiter/1 -> Speed Des(m/s)/1
  Constant8/1 -> "1 - Arm, 0 - Disarm1"/2
  "Distane To Lane (0) "/1 -> [b_n]
  Speed Selector (1)/1 -> Saturation1/1
  Speed reduction enable/1 -> Speed reduction/1
  Sliding window/1 -> [slding_window]
  ratio_ref/1 -> [ratio_ref]
  bright_ref/1 -> [bright_ref]

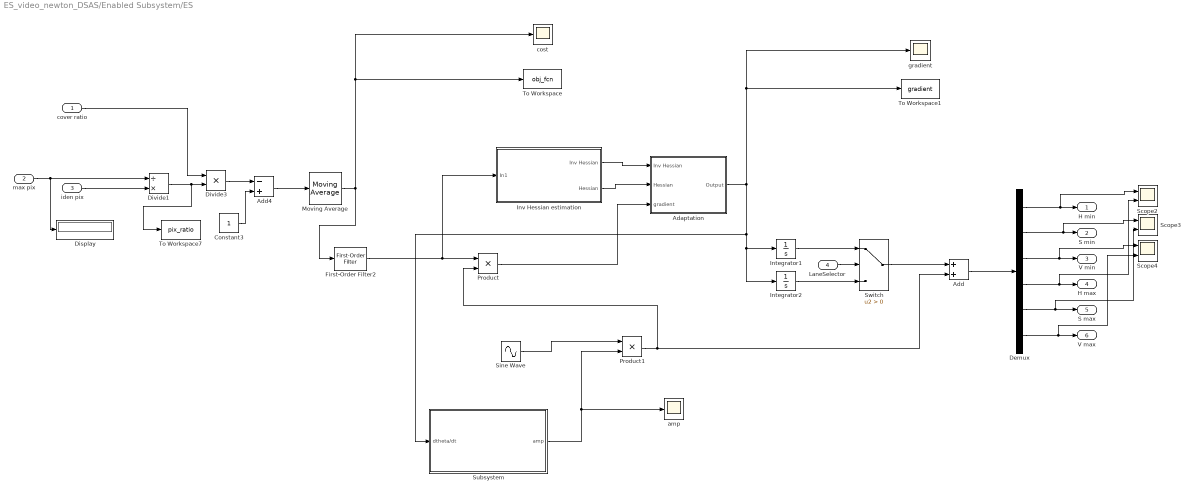
== system ES_video_newton_DSAS/Enabled Subsystem/ES ==
  "cover ratio " : Inport
  "max pix " : Inport  Port=2
  iden pix : Inport  Port=3
  LaneSelector : Inport  Port=4
  Adaptation : Subsystem
  Add : Sum
  Add4 : Sum  Inputs=-+
  Constant3 : Constant
  Demux : Demux  Outputs=6
  Display : Display
  Divide1 : Product  Inputs=/*
  Divide3 : Product  Inputs=**
  First-Order Filter2 : powerlib_meascontrol/Filters/First-Order Filter  FilterType=Highpass  Tc=30  Ts=0  Initialize=off  Vac_Init=[0, 0, 60]  Vdc_Init=0  PlotResponse=off  FreqRange="[0,  200,  1]"
  Integrator1 : Integrator  InitialCondition=[0;100;150;100;255;255]  UpperSaturationLimit=255  LowerSaturationLimit=0
  Integrator2 : Integrator  InitialCondition=[0;0;150;255;50;255]  UpperSaturationLimit=255  LowerSaturationLimit=0
  Inv Hessian estimation : Subsystem
  Moving Average : dspstat3/Moving Average  Method=Sliding window  ForgettingFactorPort=off  SpecifyWindowLength=on  WindowLength=240  ForgettingFactor=0.9  SimulateUsing=Code generation
  Product : Product
  Product1 : Product
  Scope2 : Scope  NumInputPorts=2
  Scope3 : Scope  NumInputPorts=2
  Scope4 : Scope  NumInputPorts=2
  Sine Wave : Sin  Frequency=freq  SampleTime=0
  Subsystem : Subsystem
  Switch : Switch  Criteria=u2 > Threshold
  To Workspace : ToWorkspace  VariableName=obj_fcn  SaveFormat=Timeseries  SampleTime=-1
  To Workspace1 : ToWorkspace  VariableName=gradient  SaveFormat=Timeseries  SampleTime=-1
  To Workspace7 : ToWorkspace  VariableName=pix_ratio  SaveFormat=Structure With Time  SampleTime=-1
  "amp " : Scope
  cost : Scope
  gradient : Scope
  H min : Outport  VectorParamsAs1DForOutWhenUnconnected=off
  S min : Outport  Port=2  VectorParamsAs1DForOutWhenUnconnected=off
  V min : Outport  Port=3  VectorParamsAs1DForOutWhenUnconnected=off
  H max : Outport  Port=4  VectorParamsAs1DForOutWhenUnconnected=off
  S max : Outport  Port=5  VectorParamsAs1DForOutWhenUnconnected=off
  V max : Outport  Port=6  VectorParamsAs1DForOutWhenUnconnected=off
  wires:
  Demux/1 -> Scope2/1, H min/1
  Demux/2 -> Scope3/1, S min/1
  Demux/3 -> Scope4/1, V min/1
  Demux/4 -> Scope2/2, H max/1
  Demux/5 -> Scope3/2, S max/1
  Demux/6 -> Scope4/2, V max/1
  Add/1 -> Demux/1
  "cover ratio "/1 -> Divide3/1
  iden pix/1 -> Divide1/2
  "max pix "/1 -> Display/1, Divide1/1
  Add4/1 -> Moving Average/1
  Divide1/1 -> To Workspace7/1, Divide3/2
  Divide3/1 -> Add4/1
  Constant3/1 -> Add4/2
  Moving Average/1 -> First-Order Filter2/1, To Workspace/1, cost/1
  Integrator1/1 -> Switch/1
  Integrator2/1 -> Switch/3
  Adaptation/1(Output) -> To Workspace1/1, gradient/1, Subsystem/1(dtheta/dt), Integrator2/1, Integrator1/1
  LaneSelector/1 -> Switch/2
  Switch/1 -> Add/1
  First-Order Filter2/1 -> Inv Hessian estimation/1(In1), Product/1
  Inv Hessian estimation/2(Hessian) -> Adaptation/2(Hessian)
  Inv Hessian estimation/1(Inv Hessian) -> Adaptation/1(Inv Hessian)
  Product/1 -> Adaptation/3(gradient)
  Subsystem/1(amp) -> Product1/2, "amp "/1
  Sine Wave/1 -> Product1/1
  Product1/1 -> Product/2, Add/2

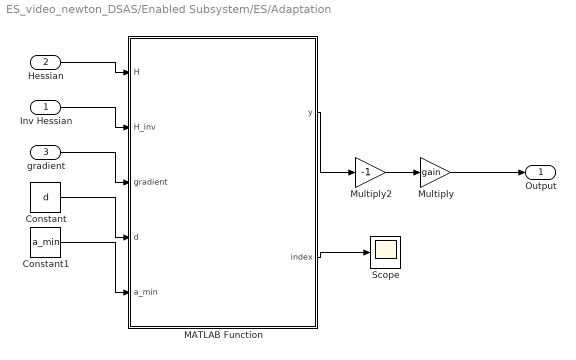
== system ES_video_newton_DSAS/Enabled Subsystem/ES/Adaptation ==
  Inv Hessian : Inport
  Hessian : Inport  Port=2
  gradient : Inport  Port=3
  Constant : Constant  Value=d
  Constant1 : Constant  Value=a_min
  MATLAB Function : MATLAB Function  TreatAsAtomicUnit=on
  Multiply : Gain  Gain=gain
  Multiply2 : Gain  Gain=-1
  Scope : Scope
  Output : Outport  VectorParamsAs1DForOutWhenUnconnected=off
  wires:
  Hessian/1 -> MATLAB Function/1(H)
  Multiply/1 -> Output/1
  MATLAB Function/1(y) -> Multiply2/1
  Inv Hessian/1 -> MATLAB Function/2(H_inv)
  gradient/1 -> MATLAB Function/3(gradient)
  Constant1/1 -> MATLAB Function/5(a_min)
  Constant/1 -> MATLAB Function/4(d)
  MATLAB Function/2(index) -> Scope/1
  Multiply2/1 -> Multiply/1

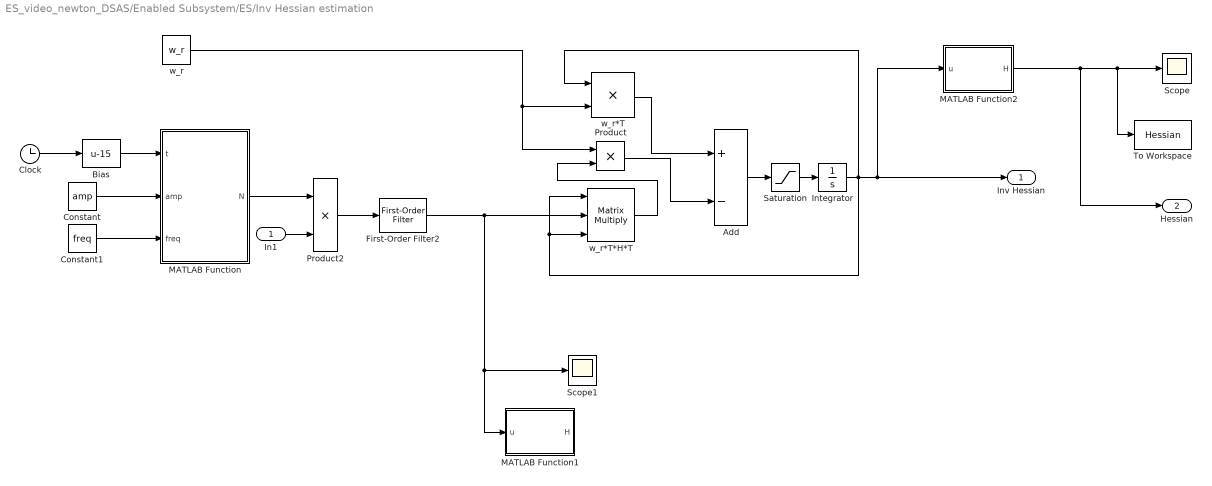
== system ES_video_newton_DSAS/Enabled Subsystem/ES/Inv Hessian estimation ==
  In1 : Inport
  Add : Sum  Inputs=+-
  Bias : Bias  Bias=-15
  Clock : Clock
      settings: Decimation=100
  Constant : Constant  Value=amp
  Constant1 : Constant  Value=freq
  First-Order Filter2 : powerlib_meascontrol/Filters/First-Order Filter  FilterType=Lowpass  Tc=15  Ts=0  Initialize=off  Vac_Init=[0 0 0]  Vdc_Init=[2;2;2;2;2;2]  PlotResponse=off  FreqRange="[0,  200,  1]"
  Integrator : Integrator  InitialCondition=IC
  MATLAB Function : MATLAB Function  TreatAsAtomicUnit=on
  MATLAB Function1 : MATLAB Function  TreatAsAtomicUnit=on
  MATLAB Function2 : MATLAB Function  TreatAsAtomicUnit=on
  Product : Product
  Product2 : Product
  Saturation : Saturate  UpperLimit=10000  LowerLimit=-10000
  Scope : Scope
  Scope1 : Scope
  To Workspace : ToWorkspace  VariableName=Hessian  SaveFormat=Timeseries  SampleTime=-1
  "w_r " : Constant  Value=w_r
  w_r*T : Product
  w_r*T*H*T : Product  Inputs=3  Multiplication=Matrix(*)
  Inv Hessian : Outport  VectorParamsAs1DForOutWhenUnconnected=off
  Hessian : Outport  Port=2  VectorParamsAs1DForOutWhenUnconnected=off
  wires:
  MATLAB Function/1(N) -> Product2/1
  In1/1 -> Product2/2
  Integrator/1 -> w_r*T*H*T/1, w_r*T*H*T/3, w_r*T/1, Inv Hessian/1, MATLAB Function2/1(u)
  w_r*T/1 -> Add/1
  Add/1 -> Saturation/1
  Clock/1 -> Bias/1
  Constant/1 -> MATLAB Function/2(amp)
  Constant1/1 -> MATLAB Function/3(freq)
  "w_r "/1 -> Product/1, w_r*T/2
  w_r*T*H*T/1 -> Product/2
  Product/1 -> Add/2
  Bias/1 -> MATLAB Function/1(t)
  MATLAB Function2/1(H) -> Hessian/1, Scope/1, To Workspace/1
  Product2/1 -> First-Order Filter2/1
  Saturation/1 -> Integrator/1
  First-Order Filter2/1 -> Scope1/1, MATLAB Function1/1(u), w_r*T*H*T/2

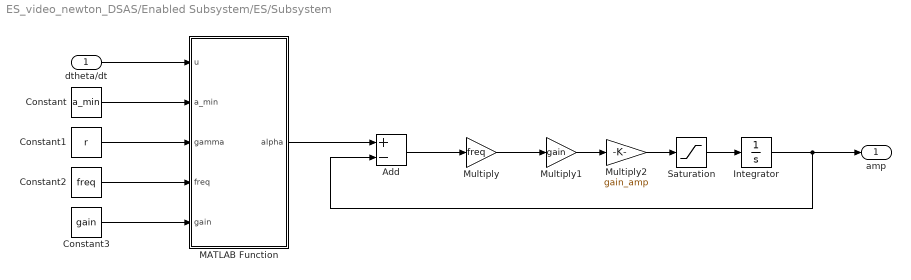
== system ES_video_newton_DSAS/Enabled Subsystem/ES/Subsystem ==
  dtheta/dt : Inport
  Add : Sum  Inputs=+-
  Constant : Constant  Value=a_min
  Constant1 : Constant  Value=r
  Constant2 : Constant  Value=freq
  Constant3 : Constant  Value=gain
  Integrator : Integrator  InitialCondition=amp
  MATLAB Function : MATLAB Function  TreatAsAtomicUnit=on
  Multiply : Gain  Gain=freq
  Multiply1 : Gain  Gain=gain
  Multiply2 : Gain  Gain=gain_amp
  Saturation : Saturate  UpperLimit=1000  LowerLimit=-1000
  amp : Outport  VectorParamsAs1DForOutWhenUnconnected=off
  wires:
  dtheta/dt/1 -> MATLAB Function/1(u)
  Constant/1 -> MATLAB Function/2(a_min)
  Constant1/1 -> MATLAB Function/3(gamma)
  Constant2/1 -> MATLAB Function/4(freq)
  Constant3/1 -> MATLAB Function/5(gain)
  MATLAB Function/1(alpha) -> Add/1
  Add/1 -> Multiply/1
  Multiply/1 -> Multiply1/1
  Multiply1/1 -> Multiply2/1
  Multiply2/1 -> Saturation/1
  Integrator/1 -> Add/2, amp/1
  Saturation/1 -> Integrator/1

== matlab function ES_video_newton_DSAS/steeringCalculation/Quick Resize1 ==
  data: u input; y output
function y = quickResize(u)

scale = 3;
    if length(size(u)) == 3
        y = u(1:scale:end, 1:scale:end, :);
    else
        y = u(1:scale:end, 1:scale:end);
    end

end

== matlab function ES_video_newton_DSAS/Enabled Subsystem/ES/Adaptation/MATLAB Function ==
  data: H input; y output; H_inv input; gradient input; d input; a_min input; index output
function [y,index] = fcn(H, H_inv, gradient, d, a_min)
y = zeros(6,1);
% gradient = gradient./(amp.^2);
for i = 1:6
    if H(1,i)*d(i,1)*a_min(i,1) > abs(gradient(i,1))
        y(i,1) = H_inv(i,:)*gradient;
        index = 1;
    else
        y(i,1) = d(i,1)*a_min(i,1)*sign(gradient(i,1));
        index = 0;
    end
end

== matlab function ES_video_newton_DSAS/MATLAB Function ==
  data: imageRGB input; imageToThreshold output; laneSelector input; imageSize output
function [imageToThreshold, imageSize]  = imageSelector(imageRGB, laneSelector)

[ROW, COL, ~] = size(imageRGB);
% imageToThreshold = uint8(zeros(ROW/2+1,COL/3,3));
if laneSelector
    imageToThreshold = imageRGB(ROW/2+1:ROW, COL*(2/3) + 1:COL, :);
else
    imageToThreshold = imageRGB(ROW/2+1:ROW, 1:COL/3, :);
end
lookupRow = 220;
imageToThreshold(1: ROW/2 - (ROW - lookupRow + 1),:,:) = 0;
imageSize = [ROW - lookupRow + 1, COL/3];

% slope_l = -0.324;
% slope2_l = -0.367;
% intercept_up_l = 145.3;
% intercept_down_l = 162.1;
% for i = 1:273
%     y_down_l = floor(slope2_l*i+intercept_down_l);
%     y_up_l = floor(slope_l*i+intercept_up_l);
%     imageToThreshold(y_up_l:y_down_l,i,:) = 0;
% end
% 
% slope_l = 0.269;
% slope2_l = 0.315;
% intercept_up_l = 58.9;
% intercept_down_l = 65.2;
% for i = 1:size(imageToThreshold,2)
%     y_down_l = floor(slope2_l*i+intercept_down_l);
%     y_up_l = floor(slope_l*i+intercept_up_l);
%     imageToThreshold(y_up_l:y_down_l,i,:) = 0;
% end

== matlab function ES_video_newton_DSAS/Enabled Subsystem/ES/Subsystem/MATLAB Function ==
  data: u input; alpha output; a_min input; gamma input; freq input; gain input
function alpha = fcn(u,a_min,gamma,freq,gain)
alpha = zeros(6,1);
a = abs(gamma./(gain.*freq).*u);
for i = 1:6
    alpha(i,1) = max(a(i,1),a_min(i,1));
end

== matlab function ES_video_newton_DSAS/Enabled Subsystem/ES/Inv Hessian estimation/MATLAB Function ==
  data: t input; N output; amp input; freq input
function N = fcn(t,amp, freq)
N = zeros(6,6);
for i = 1:6
    for j = 1:6
        if i ==j
            N(i,i) = 16/amp(i)^2*(sin(freq(i)*t)^2-1/2);
        else
            N(i,j) = 4/(amp(i)*amp(j))*sin(freq(i)*t)*sin(freq(j)*t);
        end
    end
end

== matlab function ES_video_newton_DSAS/steeringCalculation/Find slope and intercept ==
  data: Binary input; m output; b output; laneSelector input; imageSize input; pix_size output; cover_pix output; cover_ratio_bright output
function [m,... 
    b,...
    pix_size,...
    cover_pix,...
    cover_ratio_bright] = linearPolyFit(Binary, laneSelector, imageSize)

% find the shape of the incoming image
[ROW, ~] = size(Binary);

% find row, col pairs of points where pixel value is bright
[rows, cols] = find(Binary(ROW - imageSize(1) + 1:end, :) > 0);

% x is coloumns, y is max_row - rows
if laneSelector
    x = imageSize(2) - cols;
else
    x = cols;
end

y = imageSize(1) - rows;

% fit a linear polynomial to the points and grab slope, intercept
% result = polyfit(x(idx), y(idx), 1);
result = polyfit(x, y, 1);
m = result(1); 
b = result(2);


% Bright cover white lane
if laneSelector
    slope_l = 0.269;
    slope2_l = 0.315;
    intercept_up_l = 58.9;
    intercept_down_l = 65.2;
else
    slope_l = -0.324;%-0.324;
    slope2_l = -0.367;%-0.367; 
    intercept_up_l = 145.3;
    intercept_down_l = 162.1;
end

a = 5*ones(size(Binary,1),size(Binary,2));
for i = 1:size(Binary,2)
    y_down_l = floor(slope2_l*i+intercept_down_l);
    y_up_l = floor(slope_l*i+intercept_up_l);
    a(y_up_l:y_down_l,i) = 255;
end


pix_size = size(find(a==255),1);
bright = size(x,1);
% bright_ratio = bright/pix_size;

if bright == 0
    bright = 1;
end


cover_pix = size(find(a==Binary),1);
% cover_ratio = cover_pix/pix_size;
cover_ratio_bright = cover_pix/bright;
% uncover_pix = bright-cover_pix;
% uncover_ratio = uncover_pix/pix_size;
% uncover_ratio_bright = uncover_pix/bright;

% if cover_pix > 2000
%     cover_pix = 2000;
% end
% 
% pix_size = 2000;

== matlab function ES_video_newton_DSAS/Enabled Subsystem/ES/Inv Hessian estimation/MATLAB Function1 ==
  data: u input; H output
function H = fcn(u)
H = [u(1,1),u(2,2),u(3,3),u(4,4),u(5,5),u(6,6)];

== matlab function ES_video_newton_DSAS/steeringCalculation/MATLAB Function ==
  data: m input; steering output; b input; binaryShape input; gain input; laneSelector input; m_n input; b_n input
function steering = fcn(m, b, binaryShape, gain, laneSelector, m_n, b_n)
 
% y = mx + b

current_x = (binaryShape(1) - b)/m;
nominal_x = (binaryShape(1) - b_n)/m_n;
if laneSelector
    steering = -gain*(nominal_x - current_x)/binaryShape(2);
else
    steering = gain*(nominal_x - current_x)/binaryShape(2);

end

== matlab function ES_video_newton_DSAS/steeringCalculation/Quick Resize ==
  data: u input; y output
function y = quickResize(u)

scale = 3;
    if length(size(u)) == 3
        y = u(1:scale:end, 1:scale:end, :);
    else
        y = u(1:scale:end, 1:scale:end);
    end

end

== matlab function ES_video_newton_DSAS/steeringCalculation/Combine images ==
  data: laneSelector input; Binary input; RGB input; y output size=[114,274,3]; enable input; lookupRow input
function y = laneMask(laneSelector, Binary, RGB, enable, lookupRow)

y = RGB;
[ROW, COL, ~] = size(y);
[binRow, ~] = size(Binary);
binarySection = Binary(binRow-(length(lookupRow:ROW))+1:binRow,:);
if enable
    if laneSelector
        section = RGB(lookupRow:ROW, COL*(2/3) + 1:COL, :);
        y(lookupRow:ROW, ceil(COL*(2/3)) + 1:COL, 1) = ((255 - binarySection)/255).*section(:,:,1) + (binarySection).*section(:, :, 1);
        y(lookupRow:ROW, ceil(COL*(2/3)) + 1:COL, 2) = ((255 - binarySection)/255).*section(:,:,2);
        y(lookupRow:ROW, ceil(COL*(2/3)) + 1:COL, 3) = ((255 - binarySection)/255).*section(:,:,3);
    else
        section = RGB(lookupRow:ROW, 1:COL/3, :);
        y(lookupRow:ROW, 1:COL/3, 1) = ((255 - binarySection)/255).*section(:,:,1) + (binarySection).*section(:, :, 1);
        y(lookupRow:ROW, 1:COL/3, 2) = ((255 - binarySection)/255).*section(:,:,2);
        y(lookupRow:ROW, 1:COL/3, 3) = ((255 - binarySection)/255).*section(:,:,3);
    end
end

== matlab function ES_video_newton_DSAS/MATLAB Function1 ==
  data: u input; y output
function y = fcn(u)

y = u(1:340,1:end,1:end);

== matlab function ES_video_newton_DSAS/Enabled Subsystem/ES/Inv Hessian estimation/MATLAB Function2 ==
  data: u input; H output
function H = fcn(u)
H = 1./[u(1,1),u(2,2),u(3,3),u(4,4),u(5,5),u(6,6)];
